simulink model "Resetmdl_2013a"  (R2013a)
settings: Solver=ode1  StartTime=0.0  StopTime=1  RelTol=1e-3
settings Model: SimulationMode=external  Creator=uqmech  LastModifiedBy=s4358046
settings DataIOCC: SignalLoggingSaveFormat=ModelDataLogs  SignalLoggingName=sigsOut
settings OptimizationCC: InitFltsAndDblsToZero=on
settings DebuggingCC: SaveWithParameterizedLinksMsg=none  SignalResolutionControl=TryResolveAllWithWarning  SolverPrmCheckMsg=none  MultiTaskDSMMsg=warning  MultiTaskCondExecSysMsg=none  FrameProcessingCompatibilityMsg=error  StrictBusMsg=None
settings HardwareCC: ProdBitPerLong=64  ProdBitPerPointer=64  ProdIntDivRoundTo=Zero  ProdEndianess=LittleEndian  ProdWordSize=64  ProdHWDeviceType=Intel->x86-64  TargetBitPerLong=64  TargetBitPerPointer=64  TargetIntDivRoundTo=Zero  TargetEndianess=LittleEndian  TargetWordSize=64  TargetHWDeviceType=Intel->x86-64
settings RTWCC: SystemTargetFile=rtwin.tlc  TemplateMakefile=rtwin.tmf  Description=Real-Time Windows Target
settings RTWinTargetCC: TargetFcnLib=ansi_tfl_tmw.mat  TargetPreCompLibLocation=C:\Program Files\MATLAB\R2015a\toolbox\sldrt\lib\win64  CodeReplacementLibrary=C89/C90 (ANSI)  ModelReferenceCompliant=off  CompOptLevelCompliant=off

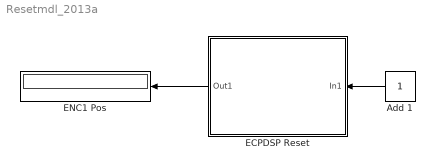
== system Resetmdl_2013a ==
  Add 1 : Constant
  ECPDSP Reset : Subsystem  mask{BaseAddr='0xC000', STime=0.001, TimeOutPer=500, HWAccess=on}
      mask prompts: BaseAddr "Base I/O Address"; STime "Sample Time (Sec)"; TimeOutPer "Timeout Period (500 ~ 2000)"; HWAccess "Hardware Access"
      mask Display: color('black');disp('ECPDSP Reset\n Will reset Dacs and Encs')
  ENC1 Pos : Display
  wires:
  Add 1/1 -> ECPDSP Reset/1(In1)
  ECPDSP Reset/1(Out1) -> ENC1 Pos/1

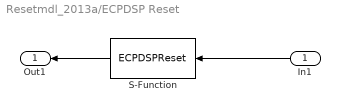
== system Resetmdl_2013a/ECPDSP Reset ==
  In1 : Inport
  S-Function : S-Function  FunctionName=ECPDSPReset  Parameters=BaseAddr,STime,TimeOutPer,HWAccess
  Out1 : Outport
  wires:
  In1/1 -> S-Function/1
  S-Function/1 -> Out1/1
